simulink model "DSHMWithHittingNewModel"  (R2013b)
settings: Solver=ode3  StartTime=0.0  StopTime=10.0  FixedStep=0.001  RelTol=1e-3
undefined symbols (not defined in the file): sigbuilder_block
settings Model: Creator=Deepak  LastModifiedBy=Deepak

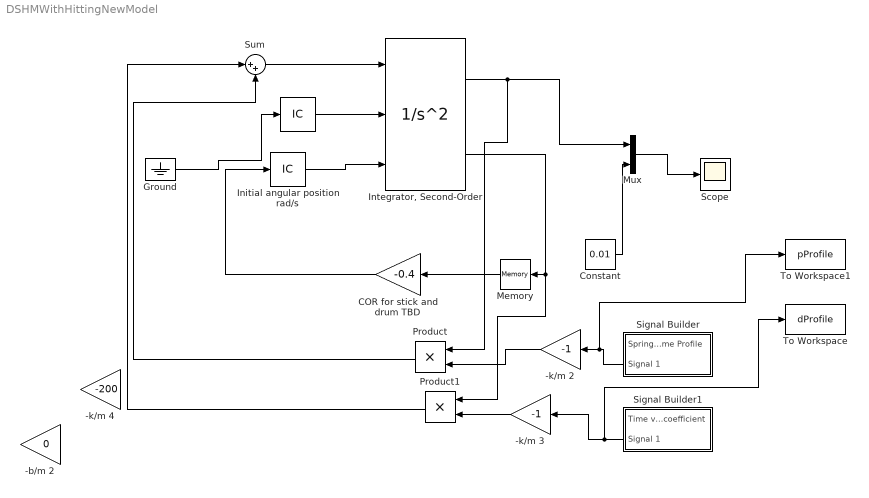
== system DSHMWithHittingNewModel ==
  " " : InitialCondition  Value=-4
  -b/m 2 : Gain  Gain=0
  -k/m 2 : Gain  Gain=-1
  -k/m 3 : Gain  Gain=-1
  -k/m 4 : Gain  Gain=-200
  COR for stick and drum TBD : Gain  Gain=-0.4
  Constant : Constant  Value=0.01
  Ground : Ground
  "Initial angular position rad/s " : InitialCondition  Value=0
  "Integrator, Second-Order" : SecondOrderIntegrator  ICSourceX=external  UpperLimitX=0.01  ICSourceDXDT=external  ReinitDXDTwhenXreachesSaturation=on
  Memory : Memory
  Mux : Mux  Inputs=2
  Product : Product
  Product1 : Product
  Scope : Scope
      settings: TimeRange=0.006119401038233385  YMin=-0.0003148134987057604  YMax=0  SaveName=ScopeData3
  Signal Builder : Subsystem  Tag=STV Subsys  LoadFcn=sigbuilder_block('load',[417.671 325.743 709.441 582.541 ]);  StartFcn=sigbuilder_block('start');  StopFcn=sigbuilder_block('stop');  ClipboardFcn=sigbuilder_block('clipboard');  mask(Sigbuilder block){}
      mask help: Simulink:masks:SigbuilderBlock_MD
      mask init:
      | if ~strcmp(get_param(bdroot(gcbh),'SimulationStatus'),'stopped') tuvar = sigbuilder_block('maskInit'); end
      settings: CopyFcn=sigbuilder_block('copy');  DeleteFcn=sigbuilder_block('delete');  ModelCloseFcn=sigbuilder_block('modelClose');  PreSaveFcn=sigbuilder_block('preSave');  PauseFcn=sigbuilder_block('pause');  ContinueFcn=sigbuilder_block('continue');  NameChangeFcn=sigbuilder_block('namechange');  OpenFcn=sigbuilder_block('open',[417.671 325.743 709.441 582.541 ]);  CloseFcn=sigbuilder_block('close');
      mask Display: plot(0, 0, 100, 100,[2, 2, 32, 32, 2], [68, 8, 8, 68, 68],[32, 2], [38, 38], [32, 19, 2],[53, 60, 44], [32, 17, 17, 2],[16, 16, 31, 31]);txt = getActiveGroup(gcbh);text(2, 100, txt,'verticalAlignment', 'top');
  Signal Builder1 : Subsystem  Tag=STV Subsys  LoadFcn=sigbuilder_block('load');  StartFcn=sigbuilder_block('start');  StopFcn=sigbuilder_block('stop');  ClipboardFcn=sigbuilder_block('clipboard');  mask(Sigbuilder block){}
      mask help: Simulink:masks:SigbuilderBlock_MD
      mask init:
      | if ~strcmp(get_param(bdroot(gcbh),'SimulationStatus'),'stopped') tuvar = sigbuilder_block('maskInit'); end
      settings: CopyFcn=sigbuilder_block('copy');  DeleteFcn=sigbuilder_block('delete');  ModelCloseFcn=sigbuilder_block('modelClose');  PreSaveFcn=sigbuilder_block('preSave');  PauseFcn=sigbuilder_block('pause');  ContinueFcn=sigbuilder_block('continue');  NameChangeFcn=sigbuilder_block('namechange');  OpenFcn=sigbuilder_block('open',[383.698 357.718 714.437 559.559 ]);  CloseFcn=sigbuilder_block('close');
      mask Display: plot(0, 0, 100, 100,[2, 2, 32, 32, 2], [68, 8, 8, 68, 68],[32, 2], [38, 38], [32, 19, 2],[53, 60, 44], [32, 17, 17, 2],[16, 16, 31, 31]);txt = getActiveGroup(gcbh);text(2, 100, txt,'verticalAlignment', 'top');
  Sum : Sum  Inputs=|++
  To Workspace : ToWorkspace  VariableName=dProfile  SampleTime=-1  SaveFormat=Structure
  To Workspace1 : ToWorkspace  VariableName=pProfile  SampleTime=-1  SaveFormat=Structure
  wires:
  COR for stick and drum TBD/1 -> "Initial angular position rad/s "/1
  "Integrator, Second-Order"/2 -> Product1/1, Memory/1
  Memory/1 -> COR for stick and drum TBD/1
  "Integrator, Second-Order"/1 -> Product/1, Mux/1
  Product/1 -> Sum/2
  Product1/1 -> Sum/1
  Sum/1 -> "Integrator, Second-Order"/1
  "Initial angular position rad/s "/1 -> "Integrator, Second-Order"/3
  " "/1 -> "Integrator, Second-Order"/2
  Ground/1 -> " "/1
  Mux/1 -> Scope/1
  Constant/1 -> Mux/2
  -k/m 2/1 -> Product/2
  -k/m 3/1 -> Product1/2
  Signal Builder/2(Signal 1) -> To Workspace1/1, -k/m 2/1
  Signal Builder1/2(Signal 1) -> To Workspace/1, -k/m 3/1

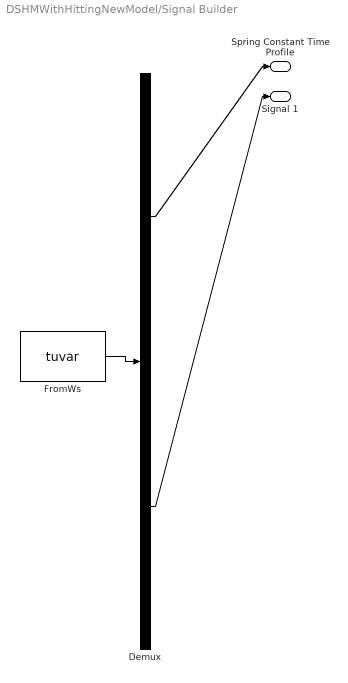
== system DSHMWithHittingNewModel/Signal Builder ==
  Demux : Demux  Tag=STV Demux  Outputs=2
  FromWs : FromWorkspace  Tag=STV FromWs  VariableName=tuvar  SampleTime=0
      SigBuilderData=|
      | common.afterFinalStr = 'Extrapolate'
      | common.sampleTime = 0
      | dataSet.timeRange = [0 10]
      | dataSet.name = 'Group 1'
      | sbobj.Groups.Name = 'Group 1'
      | sbobj.Groups.Signals(1).Name = 'Spring Constant Time Profile'
      | sbobj.Groups.Signals(1).XData = [0 10]
      | sbobj.Groups.Signals(1).YData = [0.01 980]
      | sbobj.Groups.Signals(2).Name = 'Signal 1'
      | sbobj.Groups.Signals(2).XData = [0 2 3.5 10]
      | sbobj.Groups.Signals(2).YData = [600 200 100 1]
  Spring Constant Time Profile : Outport  Tag=STV Outport
  Signal 1 : Outport  Tag=STV Outport  Port=2
  wires:
  FromWs/1 -> Demux/1
  Demux/1 -> Spring Constant Time Profile/1
  Demux/2 -> Signal 1/1

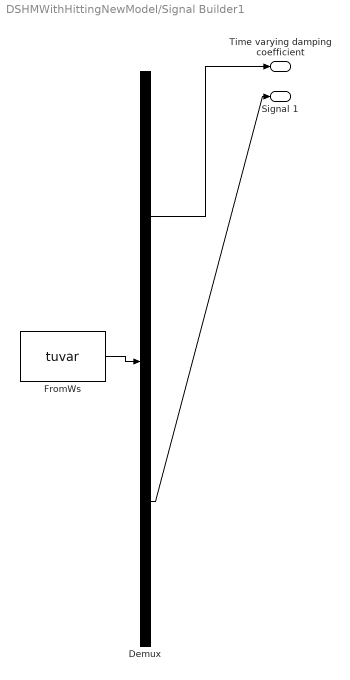
== system DSHMWithHittingNewModel/Signal Builder1 ==
  Demux : Demux  Tag=STV Demux  Outputs=2
  FromWs : FromWorkspace  Tag=STV FromWs  VariableName=tuvar  SampleTime=0
      SigBuilderData=|
      | common.afterFinalStr = 'Extrapolate'
      | common.sampleTime = 0
      | dataSet.timeRange = [0 10]
      | dataSet.name = 'Group 1'
      | sbobj.Groups.Name = 'Group 1'
      | sbobj.Groups.Signals(1).Name = 'Time varying damping coefficient'
      | sbobj.Groups.Signals(1).XData = [0 2 2 7 7 10]
      | sbobj.Groups.Signals(1).YData = [0 0 1 1 0 0]
      | sbobj.Groups.Signals(2).Name = 'Signal 1'
      | sbobj.Groups.Signals(2).XData = [0 2.3 2.8 3.1 10]
      | sbobj.Groups.Signals(2).YData = [0 0 1 1.8 1.8]
  Time varying damping coefficient : Outport  Tag=STV Outport
  Signal 1 : Outport  Tag=STV Outport  Port=2
  wires:
  FromWs/1 -> Demux/1
  Demux/1 -> Time varying damping coefficient/1
  Demux/2 -> Signal 1/1
